simulink model "sampleModel1688"  (R2023a)
settings: Solver=VariableStepAuto  StartTime=0.0  StopTime=10.0  RelTol=1e-3
libraries: hdlsllib x3
settings Model: Creator=user1  LastModifiedBy=user1

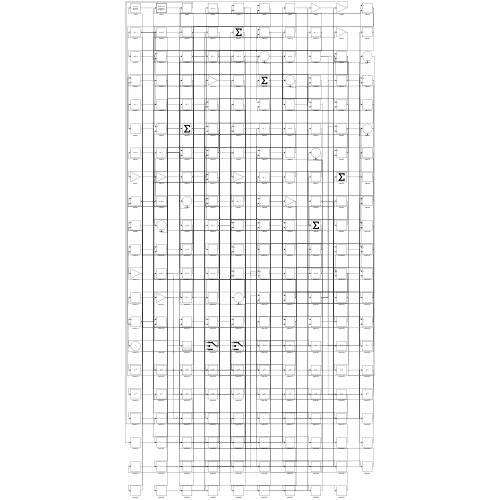
[thumbnail: Simulink's stored preview of the top-level diagram]
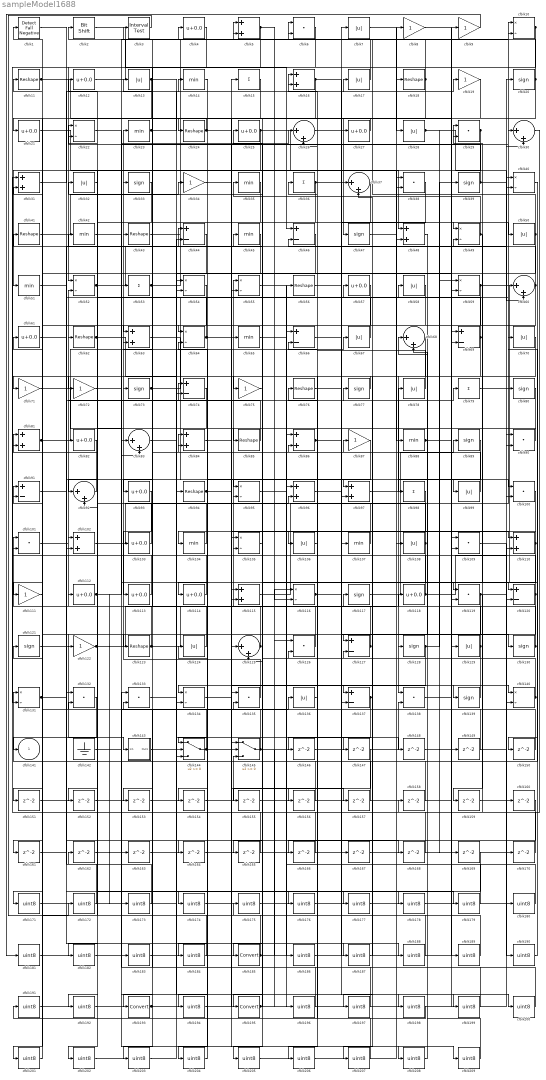
== system sampleModel1688 ==
  cfblk1 : hdlsllib/Logic and Bit Operations/Detect Fall Negative  vinit=0  OutDataTypeStr=boolean
  cfblk{10,22,40,49,52,54..55,59,64,95,105,116,131,134,140} (15 alike) : Product  Inputs=*/  RndMeth=Zero  SaturateOnIntegerOverflow=on
  cfblk{6,29,38,90,100..101,109,119,126,132..133,135,138} (13 alike) : DotProduct  OutDataTypeStr=Inherit: Inherit via internal rule
  cfblk{5,16,31,48,63,81,84,86,96..97,102,110,115} (13 alike) : Sum
  cfblk{4,12,21,25,27,57,61,82,93,103,112..114,118} (14 alike) : Bias  Bias=0.0  SaturateOnIntegerOverflow=off
  cfblk{14,23,35,42,45,51,65,88,104,107} (10 alike) : MinMax
  cfblk{7,13,17,28,32,50,58,67,70,78,99,106,108,124,129,136} (16 alike) : Abs  SaturateOnIntegerOverflow=off
  cfblk{11,18,24,41,43,56,62,76,85,94,123} (11 alike) : Reshape
  cfblk{8..9,19,34,71..72,75,87,111,122} (10 alike) : Gain
  cfblk{20,33,39,47,73,77,80,89,117,121,128,130,139} (13 alike) : Signum
  cfblk{44,46,66,69,74,91,120,127,137} (9 alike) : Sum  Inputs=+-
  cfblk{26,30,37,60,68,83,92,125} (8 alike) : Sum  Inputs=|++
  cfblk142 : Ground
  cfblk143 : Subsystem
      settings: LibrarySourceBlock=|
      | hdlsllib/Ports &
      | Subsystems/Subsystem
  cfblk144 : Switch  SaturateOnIntegerOverflow=off  InputSameDT=off
  cfblk145 : Switch  SaturateOnIntegerOverflow=off  InputSameDT=off
  cfblk{146..170} (25 alike) : Delay  SampleTime=1
  cfblk{15,36,53,79,98} (5 alike) : Sum  Inputs=+
  cfblk{171..184,186..192,194,196..209} (36 alike) : DataTypeConversion  OutDataTypeStr=uint8  SaturateOnIntegerOverflow=off  RndMeth=Floor
  cfblk185 : DataTypeConversion  SaturateOnIntegerOverflow=off  RndMeth=Floor
  cfblk193 : DataTypeConversion  SaturateOnIntegerOverflow=off  RndMeth=Floor
  cfblk195 : DataTypeConversion  SaturateOnIntegerOverflow=off  RndMeth=Floor
  cfblk2 : hdlsllib/Logic and Bit Operations/Bit Shift  mode=Shift Left Logical  N=0
  cfblk3 : hdlsllib/Logic and Bit Operations/Interval Test  IntervalClosedRight=on  uplimit=0.5  IntervalClosedLeft=on  lowlimit=-0.5  OutDataTypeStr=boolean
  cfblk141 : Outport  VectorParamsAs1DForOutWhenUnconnected=off
  wires:
  cfblk53/1 -> cfblk19/1, cfblk99/1
  cfblk117/1 -> cfblk89/1
  cfblk135/1 -> cfblk23/1
  cfblk5/1 -> cfblk52/1, cfblk116/2
  cfblk12/1 -> cfblk10/1
  cfblk121/1 -> cfblk143/1(In1)
  cfblk134/1 -> cfblk57/1
  cfblk97/1 -> cfblk79/1
  cfblk130/1 -> cfblk117/1, cfblk127/1
  cfblk87/1 -> cfblk134/1
  cfblk92/1 -> cfblk81/1
  cfblk124/1 -> cfblk101/1
  cfblk28/1 -> cfblk40/2, cfblk149/1
  cfblk19/1 -> cfblk47/1
  cfblk82/1 -> cfblk81/2
  cfblk29/1 -> cfblk51/1, cfblk123/1
  cfblk108/1 -> cfblk55/1, cfblk106/1, cfblk165/1
  cfblk59/1 -> cfblk131/1, cfblk74/2
  cfblk95/1 -> cfblk67/1
  cfblk85/1 -> cfblk52/2
  cfblk43/1 -> cfblk5/1
  cfblk111/1 -> cfblk141/1
  cfblk70/1 -> cfblk138/1
  cfblk139/1 -> cfblk32/1
  cfblk138/1 -> cfblk69/1
  cfblk21/1 -> cfblk48/1
  cfblk99/1 -> cfblk43/1
  cfblk47/1 -> cfblk18/1
  cfblk46/1 -> cfblk95/1
  cfblk79/1 -> cfblk10/2
  cfblk90/1 -> cfblk85/1
  cfblk106/1 -> cfblk86/2
  cfblk50/1 -> cfblk2/1, cfblk154/1
  cfblk17/1 -> cfblk6/1
  cfblk107/1 -> cfblk73/1
  cfblk44/1 -> cfblk111/1
  cfblk27/1 -> cfblk24/1
  cfblk10/1 -> cfblk131/2, cfblk63/1
  cfblk15/1 -> cfblk193/1
  cfblk69/1 -> cfblk29/1, cfblk3/1, cfblk146/1
  cfblk67/1 -> cfblk13/1
  cfblk72/1 -> cfblk30/1
  cfblk129/1 -> cfblk95/2, cfblk127/2
  cfblk137/1 -> cfblk87/1, cfblk156/1
  cfblk22/1 -> cfblk83/1
  cfblk52/1 -> cfblk20/1, cfblk26/1
  cfblk31/1 -> cfblk14/1
  cfblk56/1 -> cfblk27/1
  cfblk60/1 -> cfblk114/1, cfblk26/2
  cfblk73/1 -> cfblk60/1, cfblk93/1
  cfblk24/1 -> cfblk21/1, cfblk157/1
  cfblk125/1 -> cfblk62/1, cfblk63/2
  cfblk145/1 -> cfblk40/1, cfblk84/2, cfblk186/1
  cfblk120/1 -> cfblk11/1, cfblk137/2
  cfblk131/1 -> cfblk58/1, cfblk74/1
  cfblk93/1 -> cfblk113/1
  cfblk104/1 -> cfblk33/1
  cfblk114/1 -> cfblk91/1
  cfblk63/1 -> cfblk115/1
  cfblk110/1 -> cfblk104/1, cfblk197/1
  cfblk32/1 -> cfblk92/1
  cfblk112/1 -> cfblk17/1, cfblk173/1
  cfblk26/1 -> cfblk49/1
  cfblk16/1 -> cfblk50/1, cfblk75/1
  cfblk119/1 -> cfblk30/2, cfblk159/1, cfblk161/1, cfblk177/1
  cfblk84/1 -> cfblk97/1
  cfblk91/1 -> cfblk44/1
  cfblk142/1 -> cfblk136/1
  cfblk86/1 -> cfblk49/2, cfblk120/1
  cfblk105/1 -> cfblk195/1
  cfblk81/1 -> cfblk7/1, cfblk78/1
  cfblk98/1 -> cfblk137/1
  cfblk57/1 -> cfblk92/2
  cfblk115/1 -> cfblk80/1
  cfblk136/1 -> cfblk36/1
  cfblk2/1 -> cfblk46/1
  cfblk101/1 -> cfblk102/1
  cfblk103/1 -> cfblk22/1
  cfblk123/1 -> cfblk65/1, cfblk112/1
  cfblk83/1 -> cfblk44/2
  cfblk36/1 -> cfblk48/2, cfblk144/3
  cfblk64/1 -> cfblk110/1, cfblk12/1
  cfblk116/1 -> cfblk97/2, cfblk166/1
  cfblk62/1 -> cfblk134/2, cfblk6/2, cfblk119/2, cfblk208/1
  cfblk25/1 -> cfblk88/1, cfblk72/1
  cfblk122/1 -> cfblk8/1, cfblk163/1
  cfblk18/1 -> cfblk5/2, cfblk55/2, cfblk184/1
  cfblk14/1 -> cfblk64/1
  cfblk80/1 -> cfblk122/1
  cfblk128/1 -> cfblk144/1, cfblk59/1, cfblk39/1, cfblk169/1
  cfblk94/1 -> cfblk139/1, cfblk187/1
  cfblk48/1 -> cfblk98/1
  cfblk37/1 -> cfblk185/1
  cfblk77/1 -> cfblk71/1
  cfblk41/1 -> cfblk34/1
  cfblk102/1 -> cfblk96/2
  cfblk4/1 -> cfblk103/1
  cfblk34/1 -> cfblk145/1
  cfblk118/1 -> cfblk90/1, cfblk53/1
  cfblk127/1 -> cfblk82/1, cfblk84/1
  cfblk113/1 -> cfblk91/2
  cfblk78/1 -> cfblk16/1
  cfblk126/1 -> cfblk25/1
  cfblk11/1 -> cfblk129/1, cfblk107/1, cfblk164/1
  cfblk88/1 -> cfblk140/1, cfblk140/2
  cfblk7/1 -> cfblk28/1
  cfblk20/1 -> cfblk4/1, cfblk194/1
  cfblk49/1 -> cfblk35/1, cfblk119/1
  cfblk71/1 -> cfblk83/2
  cfblk140/1 -> cfblk41/1, cfblk46/2
  cfblk13/1 -> cfblk59/2, cfblk151/1
  cfblk144/1 -> cfblk77/1, cfblk31/2
  cfblk39/1 -> cfblk22/2, cfblk60/2
  cfblk89/1 -> cfblk128/1
  cfblk1/1 -> cfblk100/1
  cfblk23/1 -> cfblk16/2, cfblk168/1
  cfblk76/1 -> cfblk130/1
  cfblk146/1 -> cfblk138/2
  cfblk143/1(Out1) -> cfblk147/1
  cfblk55/1 -> cfblk148/1
  cfblk148/1 -> cfblk110/2
  cfblk149/1 -> cfblk86/1
  cfblk40/1 -> cfblk150/1
  cfblk150/1 -> cfblk1/1
  cfblk151/1 -> cfblk145/3
  cfblk58/1 -> cfblk152/1
  cfblk74/1 -> cfblk153/1
  cfblk153/1 -> cfblk96/1
  cfblk154/1 -> cfblk69/2
  cfblk75/1 -> cfblk155/1
  cfblk155/1 -> cfblk125/2
  cfblk156/1 -> cfblk101/2
  cfblk157/1 -> cfblk126/2
  cfblk30/1 -> cfblk158/1
  cfblk158/1 -> cfblk145/2
  cfblk161/1 -> cfblk102/2
  cfblk162/1 -> cfblk115/2
  cfblk163/1 -> cfblk120/2
  cfblk165/1 -> cfblk144/2
  cfblk166/1 -> cfblk31/1
  cfblk167/1 -> cfblk100/2
  cfblk168/1 -> cfblk64/2
  cfblk170/1 -> cfblk29/2
  cfblk132/1 -> cfblk171/1
  cfblk171/1 -> cfblk94/1
  cfblk3/1 -> cfblk172/1
  cfblk172/1 -> cfblk132/1
  cfblk173/1 -> cfblk132/2
  cfblk45/1 -> cfblk174/1
  cfblk174/1 -> cfblk108/1
  cfblk175/1 -> cfblk45/1
  cfblk160/1 -> cfblk176/1
  cfblk176/1 -> cfblk90/2
  cfblk177/1 -> cfblk160/1
  cfblk66/1 -> cfblk178/1
  cfblk178/1 -> cfblk118/1
  cfblk51/1 -> cfblk179/1
  cfblk179/1 -> cfblk66/1
  cfblk159/1 -> cfblk180/1
  cfblk180/1 -> cfblk66/2
  cfblk9/1 -> cfblk181/1
  cfblk181/1 -> cfblk56/1
  cfblk35/1 -> cfblk182/1
  cfblk182/1 -> cfblk9/1
  cfblk42/1 -> cfblk183/1
  cfblk183/1 -> cfblk135/1
  cfblk184/1 -> cfblk42/1
  cfblk185/1 -> cfblk175/1, cfblk167/1, cfblk116/1
  cfblk186/1 -> cfblk37/1
  cfblk187/1 -> cfblk37/2
  cfblk61/1 -> cfblk188/1
  cfblk188/1 -> cfblk162/1
  cfblk8/1 -> cfblk189/1
  cfblk189/1 -> cfblk61/1
  cfblk109/1 -> cfblk190/1
  cfblk190/1 -> cfblk70/1
  cfblk191/1 -> cfblk109/1
  cfblk169/1 -> cfblk192/1
  cfblk192/1 -> cfblk109/2
  cfblk193/1 -> cfblk170/1, cfblk125/1
  cfblk194/1 -> cfblk15/1
  cfblk195/1 -> cfblk135/2, cfblk126/1
  cfblk65/1 -> cfblk196/1
  cfblk196/1 -> cfblk105/1
  cfblk197/1 -> cfblk105/2
  cfblk133/1 -> cfblk198/1
  cfblk198/1 -> cfblk191/1
  cfblk96/1 -> cfblk199/1
  cfblk199/1 -> cfblk133/1
  cfblk152/1 -> cfblk200/1
  cfblk200/1 -> cfblk133/2
  cfblk54/1 -> cfblk201/1
  cfblk201/1 -> cfblk121/1
  cfblk33/1 -> cfblk202/1
  cfblk202/1 -> cfblk54/1
  cfblk6/1 -> cfblk203/1
  cfblk203/1 -> cfblk54/2
  cfblk38/1 -> cfblk204/1
  cfblk204/1 -> cfblk124/1
  cfblk147/1 -> cfblk205/1
  cfblk205/1 -> cfblk38/1
  cfblk100/1 -> cfblk206/1
  cfblk206/1 -> cfblk38/2
  cfblk68/1 -> cfblk207/1
  cfblk207/1 -> cfblk76/1
  cfblk208/1 -> cfblk68/1
  cfblk164/1 -> cfblk209/1
  cfblk209/1 -> cfblk68/2

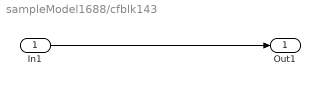
== system sampleModel1688/cfblk143 ==
  In1 : Inport
  Out1 : Outport
  wires:
  In1/1 -> Out1/1
